simulink model "ISTrain2025"  (R2025a)
settings: Solver=ode4  StartTime=0.0  StopTime=StopTime  FixedStep=StepSize  RelTol=1e-3
undefined symbols (not defined in the file or in its folder): Crr, friction_coeff, G, g, grade, kc, Ke, kf, Kt, LM, LR, m_loco, m_trail, maxID, maxIQ, maxTorque, mech_eff, Pp, R, Rr, rw
libraries: slpidlib x3
settings Model: Creator=rafae  LastModifiedBy=mmeni

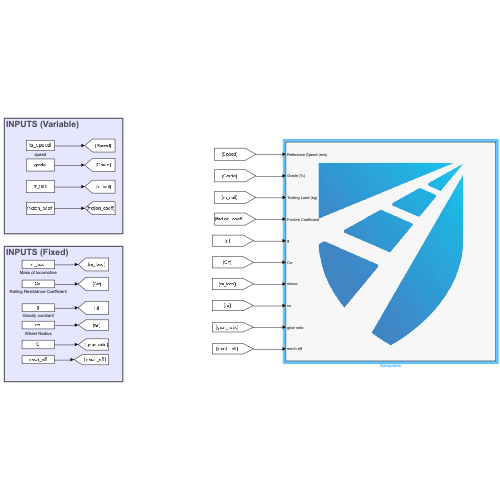
[thumbnail: Simulink's stored preview of the top-level diagram]
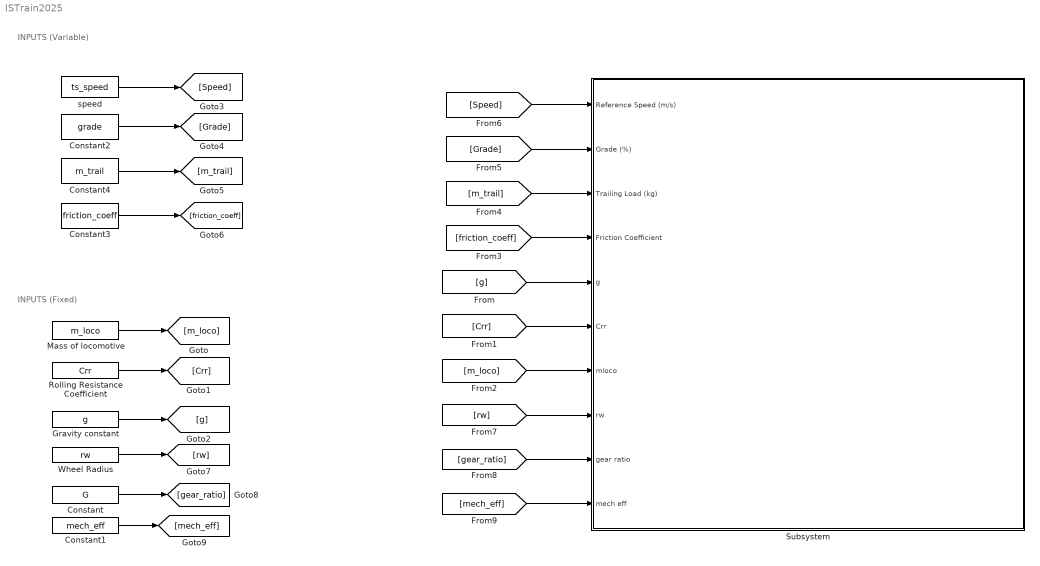
== system ISTrain2025 ==
  note: INPUTS (Variable)
  note: INPUTS (Fixed)
  Constant : Constant  Value=G
  Constant1 : Constant  Value=mech_eff
  Constant2 : Constant  Value=grade
  Constant3 : Constant  Value=friction_coeff
  Constant4 : Constant  Value=m_trail
  Gravity constant : Constant  Value=g
  Mass of locomotive : Constant  Value=m_loco
  Rolling Resistance Coefficient : Constant  Value=Crr
  Subsystem : Subsystem
      mask Display: image('ist_train_logo.jpg');
  Wheel Radius : Constant  Value=rw
  speed : FromWorkspace  VariableName=ts_speed  OutDataTypeStr=double  SampleTime=-1
  wires:
  Constant2/1 -> [Grade]
  Constant4/1 -> [m_trail]
  Mass of locomotive/1 -> [m_loco]
  Rolling Resistance Coefficient/1 -> [Crr]
  Gravity constant/1 -> [g]
  [g] -> Subsystem/5(g)
  [Crr] -> Subsystem/6(Crr)
  [m_loco] -> Subsystem/7(mloco)
  [friction_coeff] -> Subsystem/4(Friction Coefficient)
  [m_trail] -> Subsystem/3(Trailing Load (kg))
  [Grade] -> Subsystem/2(Grade (%))
  [Speed] -> Subsystem/1(Reference Speed (m/s))
  Wheel Radius/1 -> [rw]
  [rw] -> Subsystem/8(rw)
  Constant/1 -> [gear_ratio]
  [gear_ratio] -> Subsystem/9(gear ratio)
  Constant1/1 -> [mech_eff]
  [mech_eff] -> Subsystem/10(mech eff)
  Constant3/1 -> [friction_coeff]
  speed/1 -> [Speed]

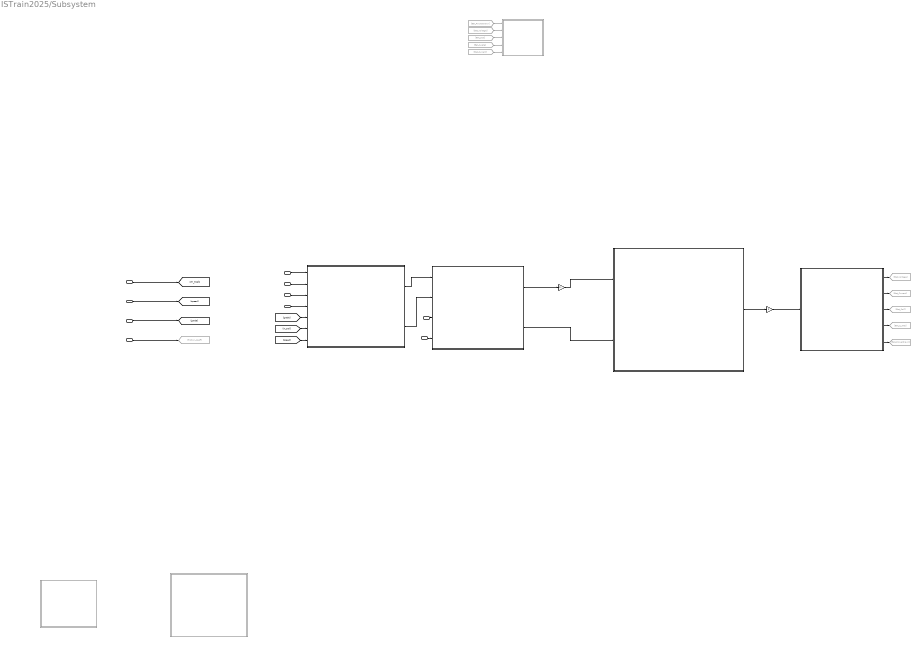
== system ISTrain2025/Subsystem ==
  note: Auxilioar Pack
  note: Drive Cycle
  note: Drivetrain
  note: Flags
  note: Controller
  note: Main Pack
  note: Motor
  Reference Speed (m/s) : Inport
  Grade (%) : Inport  Port=2
  Trailing Load (kg) : Inport  Port=3
  Friction Coefficient : Inport  Port=4
  g : Inport  Port=5
  Crr : Inport  Port=6
  mloco : Inport  Port=7
  rw : Inport  Port=8
  gear ratio : Inport  Port=9
  mech eff : Inport  Port=10
  BLDC Motor : Subsystem
      mask Display: image('motor.jpg');
  Bat_C_rate : Goto  Commented=on  GotoTag=Bat_C_rate
  Bat_Current : Goto  Commented=on  GotoTag=Bat_Current
  Bat_PowerDrawn : Goto  Commented=on  GotoTag=Bat_PowerDrawn
  Bat_SoC : Goto  Commented=on  GotoTag=Bat_SoC
  Bat_Voltage : Goto  Commented=on  GotoTag=Bat_Voltage
  Battery Alert : Subsystem  Commented=on
      mask Display: image('hazard.jpg');
  Controller : Subsystem  Commented=on
      mask Display: image('motor controller.jpeg');
  From : From  Commented=on  GotoTag=Bat_PowerDrawn
  From1 : From  Commented=on  GotoTag=Bat_Voltage
  From2 : From  Commented=on  GotoTag=Bat_SoC
  From3 : From  Commented=on  GotoTag=Bat_C_rate
  From4 : From  Commented=on  GotoTag=Bat_Current
  Gain : Gain  Gain=0.5*1.10
  Gain1 : Gain  Gain=2
  Goto3 : Goto  Commented=on  GotoTag=friction_coeff
  Primary Battery Systen : Subsystem
      mask Display: image('battery system.png');
  Secondary Battery System : Subsystem  Commented=on
      mask Display: image('battery system.png');
  Subsystem : Subsystem
      mask Display: image('gear_system.png');
  Wheel-Rail Contact : Subsystem
      mask Display: image('wheel_train.jpg');
  wires:
  Primary Battery Systen/1(Voltage) -> Bat_Voltage/1
  Primary Battery Systen/2(Current) -> Bat_Current/1
  Primary Battery Systen/3(SoC) -> Bat_SoC/1
  Primary Battery Systen/5(Power_drawn) -> Bat_PowerDrawn/1
  Primary Battery Systen/4(C_rate) -> Bat_C_rate/1
  From4/1 -> Battery Alert/5(Current)
  From3/1 -> Battery Alert/4(C_rate)
  From2/1 -> Battery Alert/3(SoC)
  From1/1 -> Battery Alert/2(Voltage)
  From/1 -> Battery Alert/1(PowerDrawn)
  Grade (%)/1 -> [grade]
  Trailing Load (kg)/1 -> [m_trail]
  Friction Coefficient/1 -> Goto3/1
  Reference Speed (m/s)/1 -> [speed]
  g/1 -> Wheel-Rail Contact/3(g)
  Crr/1 -> Wheel-Rail Contact/4(Crr)
  mloco/1 -> Wheel-Rail Contact/2(m_loco)
  ? -> ?
  [grade] -> Wheel-Rail Contact/5(grade)
  [m_trail] -> Wheel-Rail Contact/6(m_trail)
  [speed] -> Wheel-Rail Contact/7(Speed)
  rw/1 -> Wheel-Rail Contact/1(rw)
  Wheel-Rail Contact/1(T_wheel) -> Subsystem/1(T_wheel)
  Wheel-Rail Contact/2(Speed_wheel (rad/s)) -> Subsystem/2(Wheel Speed(rad/s))
  gear ratio/1 -> Subsystem/3(gear ratio)
  mech eff/1 -> Subsystem/4(mech_eff)
  Subsystem/1(Shaft Torque (Nm)) -> Gain/1
  Subsystem/2(Shaft Speed (rad/s)) -> BLDC Motor/2(Shaft Speed)
  Gain/1 -> BLDC Motor/1(Shaft Torque)
  BLDC Motor/1(P_elec) -> Gain1/1
  Gain1/1 -> Primary Battery Systen/1(P_electric)

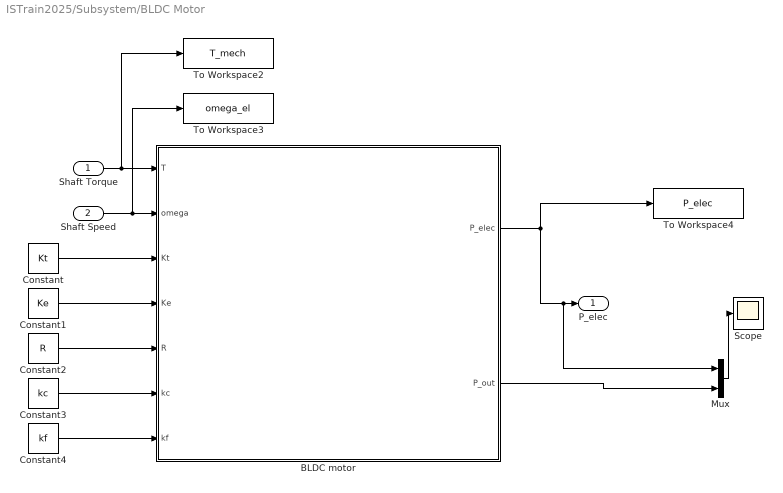
== system ISTrain2025/Subsystem/BLDC Motor ==
  Shaft Torque : Inport
  Shaft Speed : Inport  Port=2
  BLDC motor : MATLAB Function  InitFcn=""  TreatAsAtomicUnit=on
  Constant : Constant  Value=Kt
  Constant1 : Constant  Value=Ke
  Constant2 : Constant  Value=R
  Constant3 : Constant  Value=kc
  Constant4 : Constant  Value=kf
  Mux : Mux  Inputs=2
  Scope : Scope
      settings: ActiveDisplayYMinimum=-6255.3768862692459  ActiveDisplayYMaximum=11488.893381770382  DataLoggingVariableName=ScopeData7
  To Workspace2 : ToWorkspace  VariableName=T_mech  SaveFormat=Structure With Time  SampleTime=-1
  To Workspace3 : ToWorkspace  VariableName=omega_el  SaveFormat=Structure With Time  SampleTime=-1
  To Workspace4 : ToWorkspace  VariableName=P_elec  SaveFormat=Structure With Time  SampleTime=-1
  P_elec : Outport
  wires:
  Shaft Speed/1 -> To Workspace3/1, BLDC motor/2(omega)
  Shaft Torque/1 -> To Workspace2/1, BLDC motor/1(T)
  BLDC motor/1(P_elec) -> To Workspace4/1, Mux/1, P_elec/1
  Constant/1 -> BLDC motor/3(Kt)
  Constant1/1 -> BLDC motor/4(Ke)
  Constant2/1 -> BLDC motor/5(R)
  Constant3/1 -> BLDC motor/6(kc)
  Constant4/1 -> BLDC motor/7(kf)
  BLDC motor/2(P_out) -> Mux/2
  Mux/1 -> Scope/1

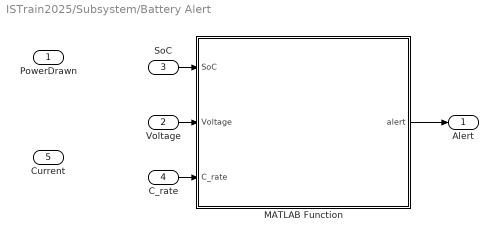
== system ISTrain2025/Subsystem/Battery Alert ==
  PowerDrawn : Inport
  Voltage : Inport  Port=2
  SoC : Inport  Port=3
  C_rate : Inport  Port=4
  Current : Inport  Port=5
  MATLAB Function : MATLAB Function  TreatAsAtomicUnit=on
  Alert : Outport
  wires:
  Voltage/1 -> MATLAB Function/2(Voltage)
  SoC/1 -> MATLAB Function/1(SoC)
  MATLAB Function/1(alert) -> Alert/1
  C_rate/1 -> MATLAB Function/3(C_rate)

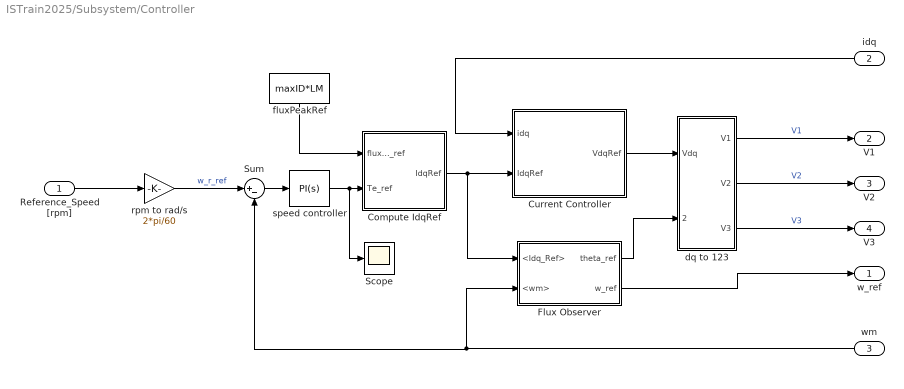
== system ISTrain2025/Subsystem/Controller ==
  Reference_Speed [rpm] : Inport
  idq : Inport  Port=2
  wm : Inport  Port=3
  Compute IdqRef : Subsystem
  Current Controller : Subsystem
  Flux Observer : Subsystem
  Scope : Scope
      settings: ActiveDisplayYMinimum=-8.125  ActiveDisplayYMaximum=73.125
  Sum : Sum  Inputs=|+-
  dq to 123 : Subsystem
  fluxPeakRef : Constant  Value=maxID*LM
  rpm to rad/s : Gain  Gain=2*pi/60
  speed controller : slpidlib/PID Controller  Controller=PI  Form=Parallel  TimeDomain=Continuous-time  UseExternalTs=off  SampleTime=-1  IntegratorMethod=Forward Euler  FilterMethod=Forward Euler  ControllerParametersSource=internal  P=50  I=100  UseKiTs=off  D=0  UseExternalDerivativeSource=off  N=100  UseFilter=on  TunerSelectOption=Transfer Function Based (PID Tuner App)  InitialConditionSource=internal  InitialConditionForIntegrator=0  InitialConditionForFilter=0  DifferentiatorICPrevScaledInput=0  ExternalReset=none  TrackingMode=off  Kt=1  LimitOutput=on  SatLimitsSource=internal  UpperSaturationLimit=maxTorque  LowerSaturationLimit=-maxTorque  LinearizeAsGain=on  AntiWindupMode=back-calculation  Kb=500  LimitIntegrator=off  UpperIntegratorSaturationLimit=inf  LowerIntegratorSaturationLimit=-inf  POutMin=[]  POutMax=[]  IOutMin=[]  IOutMax=[]  DOutMin=[]  DOutMax=[]  NOutMin=[]  NOutMax=[]  SumOutMin=[]  SumOutMax=[]  SaturationOutMin=[]  SaturationOutMax=[]  PParamMin=[]  PParamMax=[]  IParamMin=[]  IParamMax=[]  DParamMin=[]  DParamMax=[]  NParamMin=[]  NParamMax=[]  KbParamMin=[]  KbParamMax=[]  KtParamMin=[]  KtParamMax=[]  KbOutMin=[]  KbOutMax=[]  KtOutMin=[]  KtOutMax=[]  IntegratorOutMin=[]  IntegratorOutMax=[]  FilterOutMin=[]  FilterOutMax=[]  SumI1OutMin=[]  SumI1OutMax=[]  SumI2OutMin=[]  SumI2OutMax=[]  SumI3OutMin=[]  SumI3OutMax=[]  SumI4OutMin=[]  SumI4OutMax=[]  SumDOutMin=[]  SumDOutMax=[]  DifferentiatorOutMin=[]  DifferentiatorOutMax=[]  FilterDiffOutCoefMin=[]  FilterDiffOutCoefMax=[]  ReciprocalOutMin=[]  ReciprocalOutMax=[]  SumDenOutMin=[]  SumDenOutMax=[]  SumNumOutMin=[]  SumNumOutMax=[]  DivideOutMin=[]  DivideOutMax=[]  UdiffTsProdOutMin=[]  UdiffTsProdOutMax=[]  NTsProdOutMin=[]  NTsProdOutMax=[]  UintegralTsProdOutMin=[]  UintegralTsProdOutMax=[]  UngainTsProdOutMin=[]  UngainTsProdOutMax=[]  ClampingZeroOutDataTypeStr=Inherit: Inherit via back propagation  ClampingZeroOutMin=[]  ClampingZeroOutMax=[]  FilterDenConstantOutDataTypeStr=Inherit: Inherit via back propagation  FilterDenConstantOutMin=[]  FilterDenConstantOutMax=[]  PCopyOutDataTypeStr=Inherit: Inherit via back propagation  PCopyOutMin=[]  PCopyOutMax=[]  NCopyOutDataTypeStr=Inherit: Inherit via back propagation  NCopyOutMin=[]  NCopyOutMax=[]  IntegratorContinuousStateAttributes=''  IntegratorStateMustResolveToSignalObject=off  IntegratorRTWStateStorageClass=Auto  FilterContinuousStateAttributes=''  FilterStateMustResolveToSignalObject=off  FilterRTWStateStorageClass=Auto  ParallelPVariant=InternalParameters  IdealPVariant=Disabled  IVariant=InternalParameters  DVariant=Disabled  IntegratorVariant=Continuous  SatVariant=Enabled  AWVariant=BackCalculation  PCopyVariant=Disabled  TRVariant=Disabled  FdbkBlocksVariant=Forward  IdealPFdbkVariant=Disabled  SatFdbkVariant=Disabled  DerivativeFilterVariant=Disabled  NVariant=Disabled  NCopyVariant=Disabled_SignalSpec  FilterICVariant=Disabled  IntegratorICVariant=InternalICs  ExternalResetVariant=Disabled  TRSumVariant=Passthrough  SumFdbkVariant=Disabled  SumVariant=Sum_PI  TsampFilterVariant=InternalTs  TsampNgainVariant=Passthrough  TsampIntegralVariant=Disabled_SignalSpec  ExternalSaturationOutDataTypeStr=Inherit: Same as second input  DerivativeSourceVariant=Disabled  PreIntVariant=InternalPreInt
  w_ref : Outport  VectorParamsAs1DForOutWhenUnconnected=off
  V1 : Outport  Port=2  VectorParamsAs1DForOutWhenUnconnected=off
  V2 : Outport  Port=3  VectorParamsAs1DForOutWhenUnconnected=off
  V3 : Outport  Port=4  VectorParamsAs1DForOutWhenUnconnected=off
  wires:
  Compute IdqRef/1(IdqRef) -> Flux Observer/1(<Idq_Ref>), Current Controller/2(IdqRef)
  Sum/1 -> speed controller/1
  fluxPeakRef/1 -> Compute IdqRef/1(fluxdR_ref)
  dq to 123/3(V3) -> V3/1  "V3"
  wm/1 -> Sum/2, Flux Observer/2(<wm>)
  speed controller/1 -> Scope/1, Compute IdqRef/2(Te_ref)
  idq/1 -> Current Controller/1(idq)
  Reference_Speed [rpm]/1 -> rpm to rad/s/1
  dq to 123/2(V2) -> V2/1  "V2"
  dq to 123/1(V1) -> V1/1  "V1"
  rpm to rad/s/1 -> Sum/1  "w_r_ref"
  Flux Observer/2(w_ref) -> w_ref/1
  Flux Observer/1(theta_ref) -> dq to 123/2(theta_ref)
  Current Controller/1(VdqRef) -> dq to 123/1(Vdq)

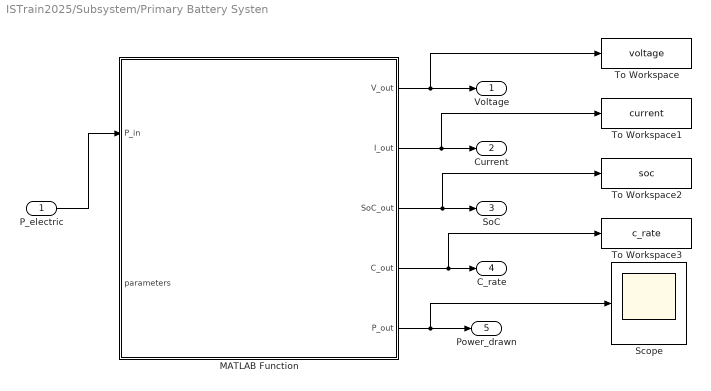
== system ISTrain2025/Subsystem/Primary Battery Systen ==
  P_electric : Inport
  MATLAB Function : MATLAB Function  TreatAsAtomicUnit=on
  Scope : Scope
      settings: ActiveDisplayYMinimum=-1  ActiveDisplayYMaximum=1  DataLoggingVariableName=ScopeData6
  To Workspace : ToWorkspace  VariableName=voltage  SaveFormat=Structure With Time  SampleTime=-1
  To Workspace1 : ToWorkspace  VariableName=current  SaveFormat=Structure With Time  SampleTime=-1
  To Workspace2 : ToWorkspace  VariableName=soc  SaveFormat=Structure With Time  SampleTime=-1
  To Workspace3 : ToWorkspace  VariableName=c_rate  SaveFormat=Structure With Time  SampleTime=-1
  Voltage : Outport
  Current : Outport  Port=2
  SoC : Outport  Port=3
  C_rate : Outport  Port=4
  Power_drawn : Outport  Port=5
  wires:
  P_electric/1 -> MATLAB Function/1(P_in)
  MATLAB Function/1(V_out) -> To Workspace/1, Voltage/1
  MATLAB Function/2(I_out) -> To Workspace1/1, Current/1
  MATLAB Function/3(SoC_out) -> To Workspace2/1, SoC/1
  MATLAB Function/4(C_out) -> To Workspace3/1, C_rate/1
  MATLAB Function/5(P_out) -> Scope/1, Power_drawn/1

== system ISTrain2025/Subsystem/Secondary Battery System ==
  In1 : Inport
  Voltage_s : Outport
  Current_s : Outport  Port=2
  SoC_s : Outport  Port=3
  C_rate_s : Outport  Port=4
  Power_drawn_s : Outport  Port=5

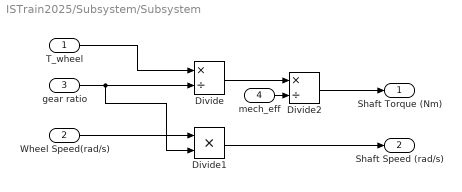
== system ISTrain2025/Subsystem/Subsystem ==
  T_wheel : Inport
  Wheel Speed(rad/s) : Inport  Port=2
  gear ratio : Inport  Port=3
  mech_eff : Inport  Port=4
  Divide : Product  Inputs=*/
  Divide1 : Product  Inputs=**
  Divide2 : Product  Inputs=*/
  Shaft Torque (Nm) : Outport
  Shaft Speed (rad/s) : Outport  Port=2
  wires:
  gear ratio/1 -> Divide1/2, Divide/2
  T_wheel/1 -> Divide/1
  Divide/1 -> Divide2/1
  Wheel Speed(rad/s)/1 -> Divide1/1
  Divide1/1 -> Shaft Speed (rad/s)/1
  mech_eff/1 -> Divide2/2
  Divide2/1 -> Shaft Torque (Nm)/1

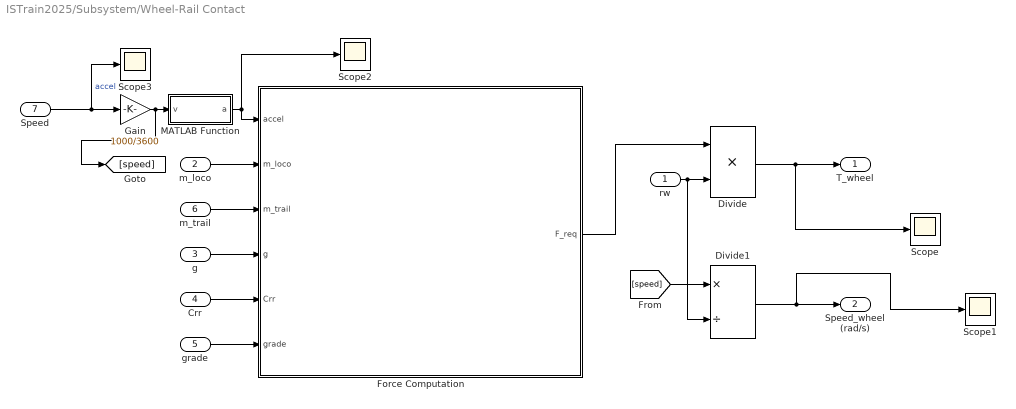
== system ISTrain2025/Subsystem/Wheel-Rail Contact ==
  rw : Inport
  m_loco : Inport  Port=2
  g : Inport  Port=3
  Crr : Inport  Port=4
  grade : Inport  Port=5
  m_trail : Inport  Port=6
  Speed : Inport  Port=7
  Divide : Product  Inputs=**
  Divide1 : Product  Inputs=*/
  Force Computation : MATLAB Function  TreatAsAtomicUnit=on
  Gain : Gain  Gain=1000/3600
  MATLAB Function : MATLAB Function  TreatAsAtomicUnit=on
  Scope{,1..3} (4 alike) : Scope
      Scope settings: ActiveDisplayYMinimum=19.793999999999862  ActiveDisplayYMaximum=57.29400000000129
      Scope1 settings: ActiveDisplayYMinimum=-1  ActiveDisplayYMaximum=1  DataLoggingVariableName=ScopeData2
      Scope2 settings: ActiveDisplayYMinimum=-0.13500000000000287  ActiveDisplayYMaximum=1.2150000000000261  DataLoggingVariableName=ScopeData4
      Scope3 settings: ActiveDisplayYMinimum=4.1736542958580607  ActiveDisplayYMaximum=7.4254364629531153  DataLoggingVariableName=ScopeData5
  T_wheel : Outport
  Speed_wheel (rad/s) : Outport  Port=2
  wires:
  g/1 -> Force Computation/4(g)
  m_loco/1 -> Force Computation/2(m_loco)
  Crr/1 -> Force Computation/5(Crr)
  grade/1 -> Force Computation/6(grade)
  m_trail/1 -> Force Computation/3(m_trail)
  MATLAB Function/1(a) -> Force Computation/1(accel), Scope2/1
  Speed/1 -> Gain/1, Scope3/1  "accel"
  rw/1 -> Divide1/2, Divide/2
  Force Computation/1(F_req) -> Divide/1
  Divide/1 -> Scope/1, T_wheel/1
  Divide1/1 -> Scope1/1, Speed_wheel (rad/s)/1
  [speed] -> Divide1/1
  Gain/1 -> [speed], MATLAB Function/1(v)

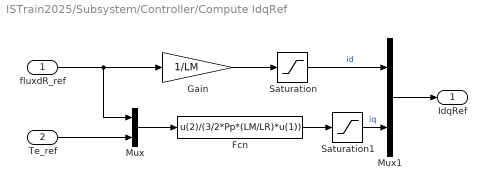
== system ISTrain2025/Subsystem/Controller/Compute IdqRef ==
  fluxdR_ref : Inport
  Te_ref : Inport  Port=2
  Fcn : Fcn  Expr=u(2)/(3/2*Pp*(LM/LR)*u(1))
  Gain : Gain  Gain=1/LM
  Mux : Mux  Inputs=2
  Mux1 : Mux  Inputs=2
  Saturation : Saturate  UpperLimit=maxID  LowerLimit=-maxID
  Saturation1 : Saturate  UpperLimit=maxIQ  LowerLimit=-maxIQ
  IdqRef : Outport  VectorParamsAs1DForOutWhenUnconnected=off
  wires:
  fluxdR_ref/1 -> Mux/1, Gain/1
  Mux/1 -> Fcn/1
  Fcn/1 -> Saturation1/1
  Gain/1 -> Saturation/1
  Mux1/1 -> IdqRef/1
  Te_ref/1 -> Mux/2
  Saturation/1 -> Mux1/1  "id"
  Saturation1/1 -> Mux1/2  "iq"

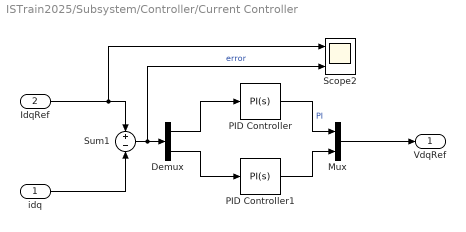
== system ISTrain2025/Subsystem/Controller/Current Controller ==
  idq : Inport
  IdqRef : Inport  Port=2
  Demux : Demux  Outputs=2
  Mux : Mux  Inputs=2
  PID Controller : slpidlib/PID Controller  Controller=PI  Form=Parallel  TimeDomain=Continuous-time  UseExternalTs=off  SampleTime=-1  IntegratorMethod=Forward Euler  FilterMethod=Forward Euler  ControllerParametersSource=internal  P=5  I=100  UseKiTs=off  D=0  UseExternalDerivativeSource=off  N=100  UseFilter=on  TunerSelectOption=Transfer Function Based (PID Tuner App)  InitialConditionSource=internal  InitialConditionForIntegrator=0  InitialConditionForFilter=0  DifferentiatorICPrevScaledInput=0  ExternalReset=none  TrackingMode=off  Kt=1  LimitOutput=on  SatLimitsSource=internal  UpperSaturationLimit=600  LowerSaturationLimit=-600  LinearizeAsGain=on  AntiWindupMode=back-calculation  Kb=1  LimitIntegrator=off  UpperIntegratorSaturationLimit=inf  LowerIntegratorSaturationLimit=-inf  POutMin=[]  POutMax=[]  IOutMin=[]  IOutMax=[]  DOutMin=[]  DOutMax=[]  NOutMin=[]  NOutMax=[]  SumOutMin=[]  SumOutMax=[]  SaturationOutMin=[]  SaturationOutMax=[]  PParamMin=[]  PParamMax=[]  IParamMin=[]  IParamMax=[]  DParamMin=[]  DParamMax=[]  NParamMin=[]  NParamMax=[]  KbParamMin=[]  KbParamMax=[]  KtParamMin=[]  KtParamMax=[]  KbOutMin=[]  KbOutMax=[]  KtOutMin=[]  KtOutMax=[]  IntegratorOutMin=[]  IntegratorOutMax=[]  FilterOutMin=[]  FilterOutMax=[]  SumI1OutMin=[]  SumI1OutMax=[]  SumI2OutMin=[]  SumI2OutMax=[]  SumI3OutMin=[]  SumI3OutMax=[]  SumI4OutMin=[]  SumI4OutMax=[]  SumDOutMin=[]  SumDOutMax=[]  DifferentiatorOutMin=[]  DifferentiatorOutMax=[]  FilterDiffOutCoefMin=[]  FilterDiffOutCoefMax=[]  ReciprocalOutMin=[]  ReciprocalOutMax=[]  SumDenOutMin=[]  SumDenOutMax=[]  SumNumOutMin=[]  SumNumOutMax=[]  DivideOutMin=[]  DivideOutMax=[]  UdiffTsProdOutMin=[]  UdiffTsProdOutMax=[]  NTsProdOutMin=[]  NTsProdOutMax=[]  UintegralTsProdOutMin=[]  UintegralTsProdOutMax=[]  UngainTsProdOutMin=[]  UngainTsProdOutMax=[]  ClampingZeroOutDataTypeStr=Inherit: Inherit via back propagation  ClampingZeroOutMin=[]  ClampingZeroOutMax=[]  FilterDenConstantOutDataTypeStr=Inherit: Inherit via back propagation  FilterDenConstantOutMin=[]  FilterDenConstantOutMax=[]  PCopyOutDataTypeStr=Inherit: Inherit via back propagation  PCopyOutMin=[]  PCopyOutMax=[]  NCopyOutDataTypeStr=Inherit: Inherit via back propagation  NCopyOutMin=[]  NCopyOutMax=[]  IntegratorContinuousStateAttributes=''  IntegratorStateMustResolveToSignalObject=off  IntegratorRTWStateStorageClass=Auto  FilterContinuousStateAttributes=''  FilterStateMustResolveToSignalObject=off  FilterRTWStateStorageClass=Auto  ParallelPVariant=InternalParameters  IdealPVariant=Disabled  IVariant=InternalParameters  DVariant=Disabled  IntegratorVariant=Continuous  SatVariant=Enabled  AWVariant=BackCalculation  PCopyVariant=Disabled  TRVariant=Disabled  FdbkBlocksVariant=Forward  IdealPFdbkVariant=Disabled  SatFdbkVariant=Disabled  DerivativeFilterVariant=Disabled  NVariant=Disabled  NCopyVariant=Disabled_SignalSpec  FilterICVariant=Disabled  IntegratorICVariant=InternalICs  ExternalResetVariant=Disabled  TRSumVariant=Passthrough  SumFdbkVariant=Disabled  SumVariant=Sum_PI  TsampFilterVariant=InternalTs  TsampNgainVariant=Passthrough  TsampIntegralVariant=Disabled_SignalSpec  ExternalSaturationOutDataTypeStr=Inherit: Same as second input  DerivativeSourceVariant=Disabled  PreIntVariant=InternalPreInt
  PID Controller1 : slpidlib/PID Controller  Controller=PI  Form=Parallel  TimeDomain=Continuous-time  UseExternalTs=off  SampleTime=-1  IntegratorMethod=Forward Euler  FilterMethod=Forward Euler  ControllerParametersSource=internal  P=5  I=100  UseKiTs=off  D=0  UseExternalDerivativeSource=off  N=100  UseFilter=on  TunerSelectOption=Transfer Function Based (PID Tuner App)  InitialConditionSource=internal  InitialConditionForIntegrator=0  InitialConditionForFilter=0  DifferentiatorICPrevScaledInput=0  ExternalReset=none  TrackingMode=off  Kt=1  LimitOutput=on  SatLimitsSource=internal  UpperSaturationLimit=600  LowerSaturationLimit=-600  LinearizeAsGain=on  AntiWindupMode=back-calculation  Kb=1  LimitIntegrator=off  UpperIntegratorSaturationLimit=inf  LowerIntegratorSaturationLimit=-inf  POutMin=[]  POutMax=[]  IOutMin=[]  IOutMax=[]  DOutMin=[]  DOutMax=[]  NOutMin=[]  NOutMax=[]  SumOutMin=[]  SumOutMax=[]  SaturationOutMin=[]  SaturationOutMax=[]  PParamMin=[]  PParamMax=[]  IParamMin=[]  IParamMax=[]  DParamMin=[]  DParamMax=[]  NParamMin=[]  NParamMax=[]  KbParamMin=[]  KbParamMax=[]  KtParamMin=[]  KtParamMax=[]  KbOutMin=[]  KbOutMax=[]  KtOutMin=[]  KtOutMax=[]  IntegratorOutMin=[]  IntegratorOutMax=[]  FilterOutMin=[]  FilterOutMax=[]  SumI1OutMin=[]  SumI1OutMax=[]  SumI2OutMin=[]  SumI2OutMax=[]  SumI3OutMin=[]  SumI3OutMax=[]  SumI4OutMin=[]  SumI4OutMax=[]  SumDOutMin=[]  SumDOutMax=[]  DifferentiatorOutMin=[]  DifferentiatorOutMax=[]  FilterDiffOutCoefMin=[]  FilterDiffOutCoefMax=[]  ReciprocalOutMin=[]  ReciprocalOutMax=[]  SumDenOutMin=[]  SumDenOutMax=[]  SumNumOutMin=[]  SumNumOutMax=[]  DivideOutMin=[]  DivideOutMax=[]  UdiffTsProdOutMin=[]  UdiffTsProdOutMax=[]  NTsProdOutMin=[]  NTsProdOutMax=[]  UintegralTsProdOutMin=[]  UintegralTsProdOutMax=[]  UngainTsProdOutMin=[]  UngainTsProdOutMax=[]  ClampingZeroOutDataTypeStr=Inherit: Inherit via back propagation  ClampingZeroOutMin=[]  ClampingZeroOutMax=[]  FilterDenConstantOutDataTypeStr=Inherit: Inherit via back propagation  FilterDenConstantOutMin=[]  FilterDenConstantOutMax=[]  PCopyOutDataTypeStr=Inherit: Inherit via back propagation  PCopyOutMin=[]  PCopyOutMax=[]  NCopyOutDataTypeStr=Inherit: Inherit via back propagation  NCopyOutMin=[]  NCopyOutMax=[]  IntegratorContinuousStateAttributes=''  IntegratorStateMustResolveToSignalObject=off  IntegratorRTWStateStorageClass=Auto  FilterContinuousStateAttributes=''  FilterStateMustResolveToSignalObject=off  FilterRTWStateStorageClass=Auto  ParallelPVariant=InternalParameters  IdealPVariant=Disabled  IVariant=InternalParameters  DVariant=Disabled  IntegratorVariant=Continuous  SatVariant=Enabled  AWVariant=BackCalculation  PCopyVariant=Disabled  TRVariant=Disabled  FdbkBlocksVariant=Forward  IdealPFdbkVariant=Disabled  SatFdbkVariant=Disabled  DerivativeFilterVariant=Disabled  NVariant=Disabled  NCopyVariant=Disabled_SignalSpec  FilterICVariant=Disabled  IntegratorICVariant=InternalICs  ExternalResetVariant=Disabled  TRSumVariant=Passthrough  SumFdbkVariant=Disabled  SumVariant=Sum_PI  TsampFilterVariant=InternalTs  TsampNgainVariant=Passthrough  TsampIntegralVariant=Disabled_SignalSpec  ExternalSaturationOutDataTypeStr=Inherit: Same as second input  DerivativeSourceVariant=Disabled  PreIntVariant=InternalPreInt
  Scope2 : Scope  NumInputPorts=2
      settings: ActiveDisplayYMinimum=-723.5766  ActiveDisplayYMaximum=3684.2345  DataLoggingVariableName=ScopeData3
  Sum1 : Sum  Inputs=+-
  VdqRef : Outport  VectorParamsAs1DForOutWhenUnconnected=off
  wires:
  IdqRef/1 -> Scope2/1, Sum1/1
  idq/1 -> Sum1/2
  PID Controller/1 -> Mux/1  "PI"
  Sum1/1 -> Scope2/2, Demux/1  "error"
  Demux/1 -> PID Controller/1
  Demux/2 -> PID Controller1/1
  PID Controller1/1 -> Mux/2
  Mux/1 -> VdqRef/1

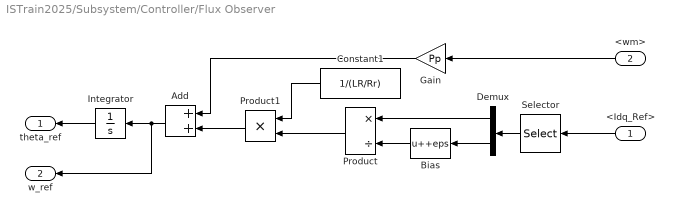
== system ISTrain2025/Subsystem/Controller/Flux Observer ==
  <Idq_Ref> : Inport
  <wm> : Inport  Port=2
  Add : Sum  Inputs=2
  Bias : Bias  Bias=+eps  SaturateOnIntegerOverflow=off
  Constant1 : Constant  Value=1/(LR/Rr)
  Demux : Demux  Outputs=2
  Gain : Gain  Gain=Pp
  Integrator : Integrator
  Product : Product  Inputs=*/
  Product1 : Product
  Selector : Selector  InputPortWidth=2  IndexOptions=Index vector (dialog)  Indices=[2 1]  OutputSizes=1
  theta_ref : Outport  VectorParamsAs1DForOutWhenUnconnected=off
  w_ref : Outport  Port=2  VectorParamsAs1DForOutWhenUnconnected=off
  wires:
  Demux/1 -> Product/1
  <wm>/1 -> Gain/1
  Constant1/1 -> Product1/1
  Selector/1 -> Demux/1
  Product1/1 -> Add/2
  Product/1 -> Product1/2
  <Idq_Ref>/1 -> Selector/1
  Add/1 -> w_ref/1, Integrator/1
  Bias/1 -> Product/2
  Demux/2 -> Bias/1
  Integrator/1 -> theta_ref/1
  Gain/1 -> Add/1

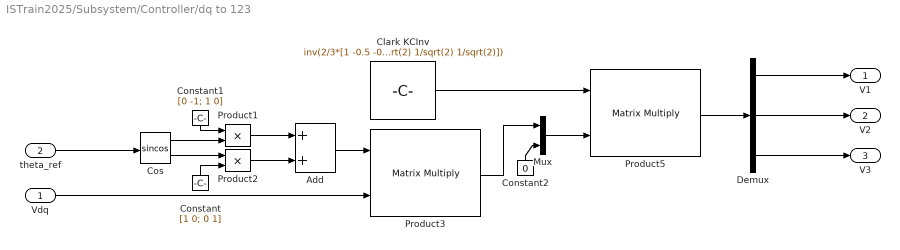
== system ISTrain2025/Subsystem/Controller/dq to 123 ==
  Vdq : Inport
  theta_ref : Inport  Port=2
  Add : Sum
  Clark KCInv : Constant  Value=inv(2/3*[1 -0.5 -0.5; 0 sqrt(3)/2 -sqrt(3)/2; 1/sqrt(2) 1/sqrt(2) 1/sqrt(2)])
  Constant : Constant  Value=[1 0; 0 1]
  Constant1 : Constant  Value=[0 -1; 1 0]
  Constant2 : Constant  Value=0
  Cos : Trigonometry  Operator=sincos
  Demux : Demux  Outputs=3
  Mux : Mux  Inputs=2
  Product1 : Product
  Product2 : Product
  Product3 : Product  Multiplication=Matrix(*)
  Product5 : Product  Multiplication=Matrix(*)
  V1 : Outport  VectorParamsAs1DForOutWhenUnconnected=off
  V2 : Outport  Port=2  VectorParamsAs1DForOutWhenUnconnected=off
  V3 : Outport  Port=3  VectorParamsAs1DForOutWhenUnconnected=off
  wires:
  Cos/1 -> Product1/2
  Constant1/1 -> Product1/1
  Product2/1 -> Add/2
  Cos/2 -> Product2/1
  Product1/1 -> Add/1
  Constant/1 -> Product2/2
  Add/1 -> Product3/1
  Product3/1 -> Mux/1
  Clark KCInv/1 -> Product5/1
  Mux/1 -> Product5/2
  Constant2/1 -> Mux/2
  Vdq/1 -> Product3/2
  Demux/1 -> V1/1
  Demux/2 -> V2/1
  Demux/3 -> V3/1
  Product5/1 -> Demux/1
  theta_ref/1 -> Cos/1

== matlab function ISTrain2025/Subsystem/Battery Alert/MATLAB Function ==
  data: SoC input; alert output; Voltage input; C_rate input
function alert = AlertZone(SoC, Voltage, C_rate)
% Throws an error if any alert condition is violated

% Thresholds
SoC_thresh = 0.10;
V_thresh   = 42;
C_thresh   = 3;

% Check conditions
if SoC < SoC_thresh
    error('ALERT: State of Charge dropped below 10%% (SoC = %.2f)', SoC);
elseif Voltage < V_thresh
    error('ALERT: Voltage dropped below minimum threshold (Voltage = %.2f V)', Voltage);
elseif C_rate > C_thresh
    error('ALERT: C-rate exceeded safe limit (C_rate = %.2f)', C_rate);
end

% No alert
alert = 0;
end

== matlab function ISTrain2025/Subsystem/Primary Battery Systen/MATLAB Function ==
  data: P_in input; V_out output; I_out output; SoC_out output; C_out output; P_out output; parameters input
function [V_out, I_out, SoC_out, C_out, P_out] = batteryModelFcn(P_in,parameters)
%#codegen
persistent SoC V_RC
dt = 0.001;

% Initialize persistent states
if isempty(SoC)
    SoC = 1;           % Start fully charged
end
if isempty(V_RC)
    V_RC = 0;          % RC voltage
end

% Battery configuration: 2 batteries in parallel
usable_capacity_Ah = 2 * 100 * 0.8;  % 160Ah usable
pack_voltage_nom = 25.6;             % Nominal voltage per battery
Q_total = usable_capacity_Ah * 3600; % Total charge in Coulombs

% Internal resistance model
R0 = 0.015;   % Ohms
R1 = 0.004;   % Ohms
C1 = 1500;    % Farads

voc_min = 22; % Minimum allowed terminal voltage

% SoC to Voc lookup
soc_points = linspace(0,1,11);
voc_points = [22.0 24.0 25.0 25.5 25.9 26.2 26.5 26.9 27.5 28.3 29.2];
Voc = interp1(soc_points, voc_points, SoC, 'linear','extrap');

% If SoC or voltage too low, shut off
if SoC <= 0.1
    I = 0;
    V_terminal = voc_min;
    P_out = 0;
else
    I = P_in / max(Voc, 1e-3);
end

% Max discharge current: 2 batteries × 100A = 200A
if I > 200
    I = 200;
    P_out = I * Voc;
else
    P_out = P_in;
end

% RC circuit dynamics
dV_RC = (-V_RC + I * R1) / (R1 * C1) * dt;
V_RC = V_RC + dV_RC;

% Terminal voltage calculation
V_terminal = Voc - I * R0 - V_RC;

% Voltage cutoff enforcement
if V_terminal < voc_min
    V_terminal = voc_min;
    I = 0;
    P_out = 0;
end

% SoC update
dQ = I * dt;
Q_used = (1 - SoC) * Q_total + dQ;
SoC = max(0, 1 - Q_used / Q_total);

% Outputs
V_out = V_terminal;
I_out = I;
SoC_out = SoC;
C_out = I / usable_capacity_Ah;
end

== matlab function ISTrain2025/Subsystem/Wheel-Rail Contact/MATLAB Function ==
  data: v input; a output
function a = diff_accel(v)
  % v is the current speed [m/s]
  persistent v_last
  if isempty(v_last)
    v_last = v;
  end
  a = (v - v_last) / 0.1;   % StepSize must be in base workspace
  v_last = v;
end

== matlab function ISTrain2025/Subsystem/Wheel-Rail Contact/Force Computation ==
  data: accel input; m_loco input; m_trail input; F_req output; g input; Crr input; grade input
function F_req = Force_Computation(accel, m_loco, m_trail, g, Crr, grade)

a=accel;
m_total=m_trail+m_loco;

F_grade = m_total * g * grade;  % grade
F_rr    = m_total * g * Crr;% rolling
F_a=m_total*a; % Force due to a imposed acceleration
F_req   = F_grade + F_rr+F_a;
end

== matlab function ISTrain2025/Subsystem/BLDC Motor/BLDC motor ==
  data: T input; P_elec output; omega input; Kt input; Ke input; R input; kc input; kf input; P_out output
function [P_elec,P_out]  = calc_elec_power(T, omega, Kt,Ke,R,kc,kf)
  %This function calculates the eletrical power needed for a given
  %mechanical power and a given motor

  % INPUTS:
  %T-Shaft Torque (N.m)
  %omega-Shaft speed (rads-1)
  % motor.Kt  – torque constant [Nm/A]
  % motor.Ke  – EMF constant [V·s/rad]
  % motor.R   – phase resistance [Ohm]
  % motor.kc  – core loss coeff (optional)
  % motor.kf  – friction coeff (optional)

  %OUTPUTS:

  %P_elec-Eletrical Power
  %eff-Motor efficiency
  
  % Phase current from torque
  I_phase   = T / Kt;
  
  % Back-EMF
  E = Ke * omega;
  
  
  % Copper losses
  P_cu = 3 * R * I_phase^2;
  
  % Core losses 
  P_core = kc * omega^2;
  
  % Friction/windage 
  P_fm   = kf * omega;
  
  % Electrical input power
  P_elec = T*omega  + P_cu + P_core + P_fm; % Electrical power
  P_out = T*omega;
  %eff= P_elec/P_mech; % Motor efficiency
end
